simulink model "Use_C_Code_in_simulink_v2"  (R2019b)
settings: Solver=FixedStepAuto  StartTime=0.0  StopTime=5/100  FixedStep=Ts  RelTol=1e-3
InitFcn:
  | fs=1e6; %100kHz
  | Ts=1/fs;
libraries: sfundemos x1, simulink x1
settings Model: Creator=W002220B  LastModifiedBy=W002220B

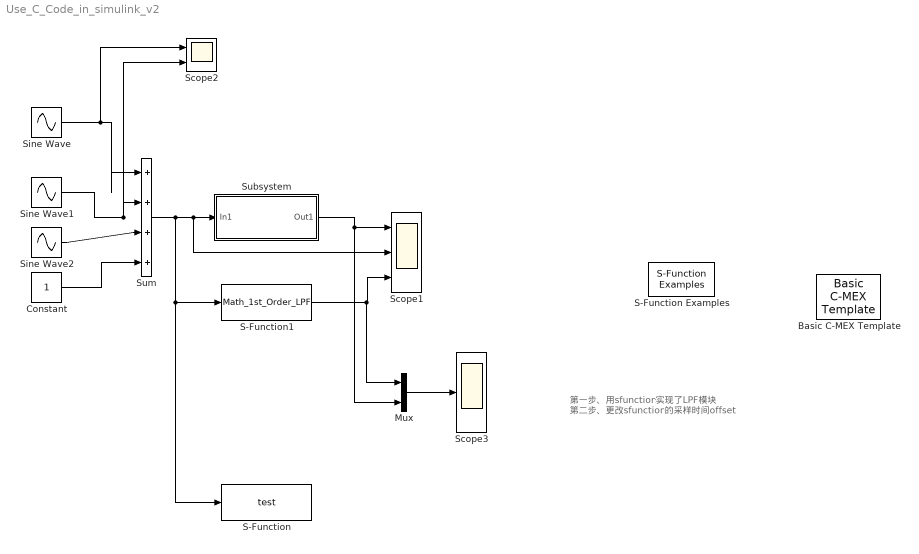
== system Use_C_Code_in_simulink_v2 ==
  note: 第一步、用sfunction实现了LPF模块
      | 第二步、更改sfunction的采样时间offset
  "Basic C-MEX Template " : sfundemos/C-file S-functions/Basic C-MEX Template   a=[]
  Constant : Constant
  Mux : Mux  Inputs=2
  S-Function : S-Function  FunctionName=test  SFunctionDeploymentMode=off  EnableBusSupport=off
  S-Function Examples : simulink/User-Defined Functions/S-Function Examples
      settings: SourceProductName=Simulink  SourceProductBaseCode=SL
  S-Function1 : S-Function  FunctionName=Math_1st_Order_LPF  Parameters=1/(2*pi*100),[10*Ts Ts]  SFunctionDeploymentMode=off  EnableBusSupport=off
  Scope1 : Scope  NumInputPorts=3
  Scope2 : Scope  NumInputPorts=2
  Scope3 : Scope
  Sine Wave : Sin  Frequency=100*2*pi  SampleTime=Ts
  Sine Wave1 : Sin  Frequency=1000*2*pi  SampleTime=Ts
  Sine Wave2 : Sin  Frequency=1e4*2*pi  SampleTime=Ts
  Subsystem : Subsystem  mask{Tf=1/(2*pi*100), Tsample=Ts}
      mask prompts: Tf "Filter Time(seconds)"; Tsample "Sample Time(seconds)"
      mask DialogControl DescTextVar Prompt: Low Pass Filter User Defined
  Sum : Sum  Inputs=|++++
  wires:
  Sine Wave/1 -> Scope2/1, Sum/1
  Sine Wave1/1 -> Scope2/2, Sum/2
  Sine Wave2/1 -> Sum/3
  Constant/1 -> Sum/4
  Sum/1 -> S-Function/1, S-Function1/1, Scope1/2, Subsystem/1(In1)
  Subsystem/1(Out1) -> Mux/2, Scope1/1
  S-Function1/1 -> Mux/1, Scope1/3
  Mux/1 -> Scope3/1

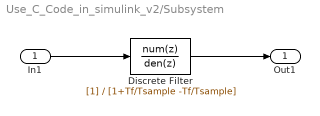
== system Use_C_Code_in_simulink_v2/Subsystem ==
  In1 : Inport
  Discrete Filter : DiscreteFilter  Denominator=[1+Tf/Tsample -Tf/Tsample]  SampleTime=Tsample
  Out1 : Outport
  wires:
  In1/1 -> Discrete Filter/1
  Discrete Filter/1 -> Out1/1
